simulink model "FE11_Telemetry_Data_Analysis"  (R2023b)
settings: Solver=VariableStepAuto  StartTime=0.0  StopTime=2618.70000000000  RelTol=1e-3
settings Model: Creator=salaz  LastModifiedBy=salaz

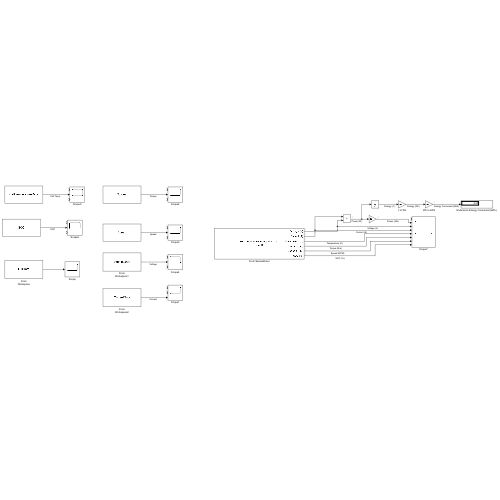
[thumbnail: Simulink's stored preview of the top-level diagram]
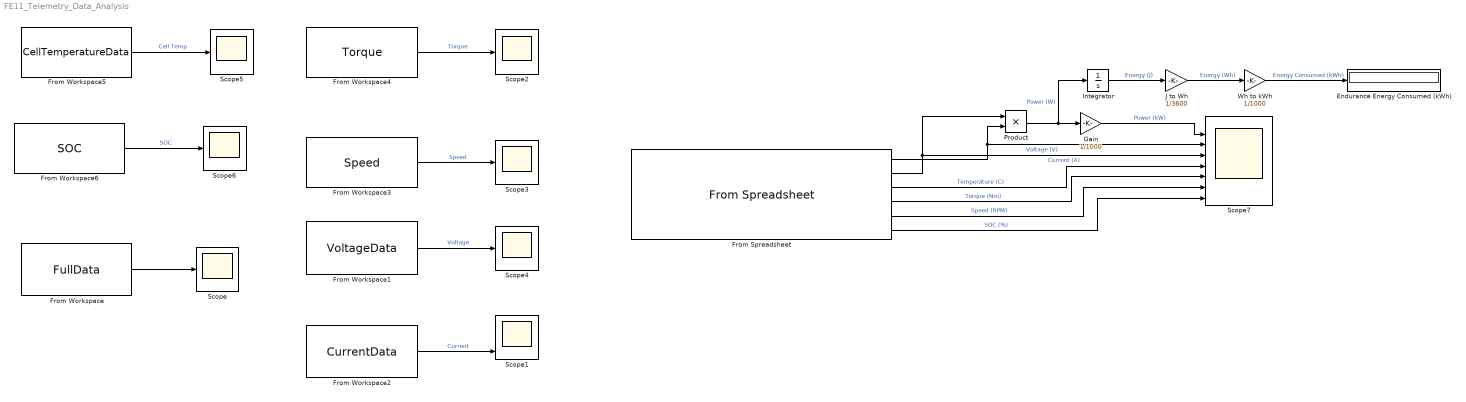
== system FE11_Telemetry_Data_Analysis ==
  "Endurance Energy Consumed (kWh) " : Display
  From Workspace : FromWorkspace  VariableName=FullData
  From Workspace1 : FromWorkspace  VariableName=VoltageData
  From Workspace2 : FromWorkspace  VariableName=CurrentData
  From Workspace3 : FromWorkspace  VariableName=Speed
  From Workspace4 : FromWorkspace  VariableName=Torque
  From Workspace5 : FromWorkspace  VariableName=CellTemperatureData
  From Workspace6 : FromWorkspace  VariableName=SOC
  From Spreadsheet : FromSpreadsheet  FileName=FE11 Endurance Full Data V2.xlsx
  Gain : Gain  Gain=1/1000
  Integrator : Integrator
  J to Wh : Gain  Gain=1/3600
  Product : Product
  Scope : Scope
  Scope{1..6} (6 alike) : Scope  NumInputPorts=3
  Scope7 : Scope  NumInputPorts=8
  Wh to kWh : Gain  Gain=1/1000
  wires:
  From Workspace/1 -> Scope/1
  From Workspace1/1 -> Scope4/2  "Voltage"
  From Workspace2/1 -> Scope1/3  "Current"
  From Workspace3/1 -> Scope3/2  "Speed"
  From Workspace4/1 -> Scope2/2  "Torque"
  From Workspace5/1 -> Scope5/2  "Cell Temp"
  From Workspace6/1 -> Scope6/2  "SOC"
  From Spreadsheet/1 -> Product/2, Scope7/3  "Voltage (V)"
  From Spreadsheet/2 -> Product/1, Scope7/4  "Current (A)"
  From Spreadsheet/3 -> Scope7/5  "Temperature (C)"
  From Spreadsheet/4 -> Scope7/6  "Torque (Nm)"
  From Spreadsheet/5 -> Scope7/7  "Speed (RPM)"
  From Spreadsheet/6 -> Scope7/8  "SOC (%)"
  Product/1 -> Integrator/1, Gain/1  "Power (W)"
  Gain/1 -> Scope7/2  "Power (kW)"
  Integrator/1 -> J to Wh/1  "Energy (J)"
  J to Wh/1 -> Wh to kWh/1  "Energy (Wh)"
  Wh to kWh/1 -> "Endurance Energy Consumed (kWh) "/1  "Energy Consumed (kWh)"
